simulink model "UdpSigSocket_Example"  (R2013a)
settings: Solver=ode45  StartTime=0.0  StopTime=inf  RelTol=1e-3
settings Model: Creator=jsUni  LastModifiedBy=jsUni

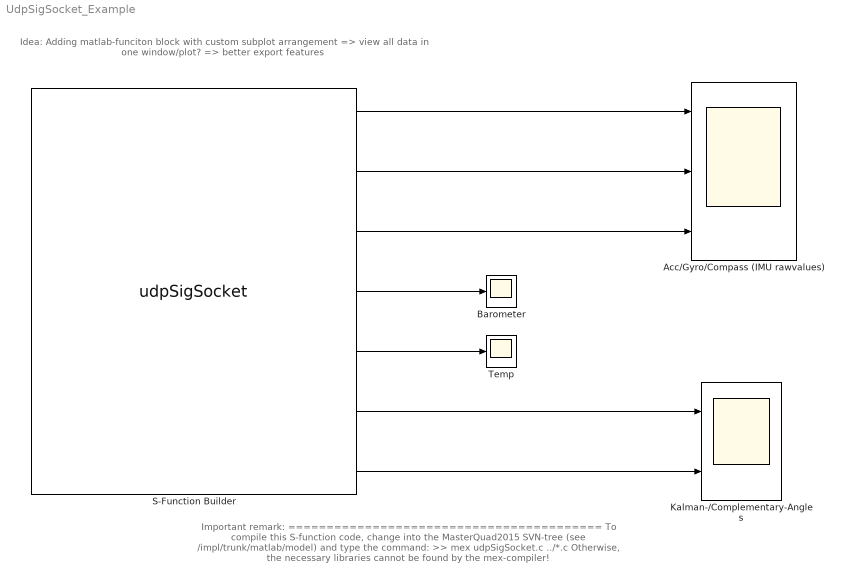
== system UdpSigSocket_Example ==
  note: Important remark:
      | =========================================
      |  To compile this S-function code, change into the MasterQuad2015
      | SVN-tree (see /impl/trunk/matlab/model) and type the command:
      | >> mex udpSigSocket.c ../*.c
      |
      | Otherwise, the necessary libraries cannot be found by the mex-compiler!
  note: Idea:
      | Adding matlab-funciton block with custom
      | subplot arrangement
      | => view all data in one window/plot? => better export features
  Acc/Gyro/Compass (IMU rawvalues) : Scope  NumInputPorts=3
      settings: YMin=-45~-5~-5  YMax=10~5~5
  Barometer : Scope
      settings: YMin=976.55  YMax=977.2  SaveName=ScopeData3
  Kalman-/Complementary-Angles : Scope  NumInputPorts=2
      settings: YMin=-175~-5  YMax=175~5  SaveName=ScopeData5
  S-Function Builder : S-Function  InitFcn=try, set_param(gcb,'FunctionName','udpSigSocket'), end  FunctionName=udpSigSocket  Parameters=0.1,5000  SFunctionModules=udpSigSocket_wrapper  EnableBusSupport=off  mask(S-Function Builder){}
      mask help: Simulink:masks:SFunctionBuilder_MD
      mask init:
      | val = [[.9  0.75 0.75 1 1 .9 .9 1]',[1 1 0.75 0.75 .9 .9 1 .9]'];try , sys = get_param(gcb,'SfunBuilderFcnName');if isempty(sys), sys = get_param(gcb,'FunctionName'); end,catch, sys = get_param(gcb,'FunctionName'); end
      settings: CopyFcn=set_param(gcbh,'LinkStatus','none')  PreSaveFcn=try, set_param(gcb,'FunctionName','udpSigSocket'), end  OpenFcn=sfunctionwizard(gcbh)
      mask Display: plot(val(:,1),val(:,2)),disp(sys), port_label('output',1,'Raw_Accelerometer_xyz'), port_label('output',2,'Raw_Gyrometer_rpy'), port_label('output',3,'Raw_Compass_xyz'), port_label('output',4,'Raw_Barometer_z'), port_label('output',5,'Raw_Temperature'), port_label('output',6,'Kalman_Angles_rpy'), port_label('output',7,'Complementary_Angles_rpy')
  Temp : Scope
      settings: YMin=32.2  YMax=32.29  SaveName=ScopeData4
  wires:
  S-Function Builder/3 -> Acc/Gyro/Compass (IMU rawvalues)/3
  S-Function Builder/2 -> Acc/Gyro/Compass (IMU rawvalues)/2
  S-Function Builder/1 -> Acc/Gyro/Compass (IMU rawvalues)/1
  S-Function Builder/5 -> Temp/1
  S-Function Builder/4 -> Barometer/1
  S-Function Builder/6 -> Kalman-/Complementary-Angles/1
  S-Function Builder/7 -> Kalman-/Complementary-Angles/2
